simulink model "dummy2"  (R2018b)
settings: Solver=FixedStepDiscrete  StartTime=0.0  StopTime=10  FixedStep=0.2  RelTol=1e-3
undefined symbols (not defined in the file): eyen, n, xmin
settings Model: Creator=bradyplanden  LastModifiedBy=bradyplanden
settings OptimizationCC: DefaultParameterBehavior=Inlined
settings SFSimCC: SimCustomHeaderCode="#include \"dummy.h\""  SimUserSources=dummy.c  SimUserIncludeDirs=/usr/lib  SimUserLibraries=libblas.dylib liblapack.dylib  SimUseLocalCustomCode=off  SimAnalyzeCustomCode=on
settings RTWCC: GenerateReport=on  RTWUseLocalCustomCode=off  RTWUseSimCustomCode=on  CustomHeaderCode="#include \"dummy.h\""  CustomInclude=/usr/lib  CustomSource=dummy.c  CustomLibrary=libblas.dylib liblapack.dylib  LaunchReport=on
settings CodeAppCC: ForceParamTrailComments=on  StateflowObjectComments=on  MATLABSourceComments=on
settings GRTTargetCC: TargetLangStandard=C89/C90 (ANSI)

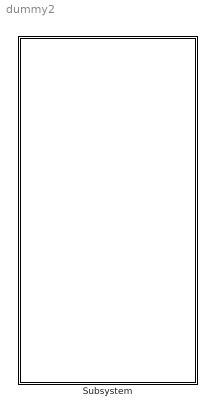
== system dummy2 ==
  Subsystem : Subsystem

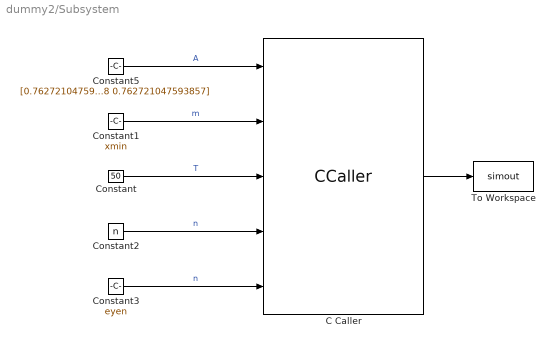
== system dummy2/Subsystem ==
  C Caller : CCaller  FunctionName=dummy2  PortSpecificationStruct="%)30     .    Z @   8    (     @         %    \"     8    !     0         %  0 \"0    $    V    07)G3F%M90  4&]R=$YA;64 4V-O<&4     26YD97@     5'EP90      4VEZ90         .    ,     8    (    !          %    \"     $    #     0         0  , ;W5T  X    P    !@    @    $          4    (     0    ,    !         !   P!O=70 #@   #@    &    \"     0         !0    @    !    !@    $         $     8   !/=7 ...(+2691 chars)"
  Constant : Constant  Value=50  OutDataTypeStr=Inherit: Inherit via back propagation  SampleTime=-1
  Constant1 : Constant  Value=xmin  OutDataTypeStr=Inherit: Inherit via back propagation  SampleTime=-1
  Constant2 : Constant  Value=n  OutDataTypeStr=Inherit: Inherit via back propagation  SampleTime=-1
  Constant3 : Constant  Value=eyen  OutDataTypeStr=Inherit: Inherit via back propagation  SampleTime=-1
  Constant5 : Constant  Value=|  OutDataTypeStr=Inherit: Inherit via back propagation  SampleTime=-1
      | [0.762721047593857	0.114882546593898	0.00247654474066823	2.09380749408769e-05	9.42229417535085e-08	2.63060135287668e-10	0.459613939727602	0.0198131117128797	0.000251260056028671	1.50757506761672e-06	5.26123024735364e-09	1.19993006342024e-11
      | 0.114882546593898	0.765197592334525	0.114903484668839	0.00247663896360998	2.09383380010122e-05	9.42229417535096e-08	0.0198131117128796	0.459865199783630	0.0198146192879473	0.000251265317258919	1.50758706691736e-06	5.26123024735407e-09
      | 0.00247654474066823	0.114903484668839	0.765197686557466	0.114903484931899	0.00247663896360999	2.09380749408770e-05	0.000251260056028671	0.0198146192879473	0.459865205044861	0.0198146192999466	0.000251265317258919	1.50757506761673e-06
      | 2.09380749408769e-05	0.00247663896360998	0.114903484931899	0.765197686557467	0.114903484668839	0.00247654474066823	1.50757506761672e-06	0.000251265317258918	0.0198146192999466	0.459865205044861	0.0198146192879473	0.000251260056028672
      | 9.42229417535087e-08	2.09383380010122e-05	0.00247663896360998	0.114903484668839	0.765197592334525	0.114882546593898	5.26123024735378e-09	1.50758706691736e-06	0.000251265317258919	0.0198146192879473	0.459865199783631	0.0198131117128796
      | 2.63060135287738e-10	9.42229417535093e-08	2.09380749408769e-05	0.00247654474066823	0.114882546593898	0.762721047593857	1.19993006342118e-11	5.26123024735394e-09	1.50757506761673e-06	0.000251260056028671	0.0198131117128797	0.459613939727602
      | -0.899414767742325	0.420238976357871	0.0193120991758899	0.000248250167123685	1.49706460642265e-06	5.23723164608530e-09	0.762721047593857	0.114882546593898	0.00247654474066823	2.09380749408769e-05	9.42229417535083e-08	2.63060135287700e-10
      | 0.420238976357871	-0.880102668566434	0.420487226524995	0.0193135962404963	0.000248255404355332	1.49706460642266e-06	0.114882546593898	0.765197592334525	0.114903484668839	0.00247663896360998	2.09383380010123e-05	9.42229417535099e-08
      | 0.0193120991758899	0.420487226524995	-0.880101171501828	0.420487231762227	0.0193135962404964	0.000248250167123686	0.00247654474066823	0.114903484668839	0.765197686557467	0.114903484931899	0.00247663896360999	2.09380749408770e-05
      | 0.000248250167123685	0.0193135962404963	0.420487231762227	-0.880101171501828	0.420487226524995	0.0193120991758899	2.09380749408769e-05	0.00247663896360998	0.114903484931899	0.765197686557467	0.114903484668839	0.00247654474066823
      | 1.49706460642265e-06	0.000248255404355331	0.0193135962404963	0.420487226524995	-0.880102668566434	0.420238976357871	9.42229417535088e-08	2.09383380010122e-05	0.00247663896360998	0.114903484668839	0.765197592334525	0.114882546593898
      | 5.23723164608547e-09	1.49706460642265e-06	0.000248250167123685	0.0193120991758899	0.420238976357872	-0.899414767742325	2.63060135287715e-10	9.42229417535098e-08	2.09380749408769e-05	0.00247654474066823	0.114882546593898	0.762721047593857]
  To Workspace : ToWorkspace  VariableName=simout  SaveFormat=Timeseries  SampleTime=-1
      settings: Decimation=4  Save2DSignal=2-D array (concatenate along first dimension)
  wires:
  Constant5/1 -> C Caller/1  "A"
  Constant2/1 -> C Caller/4  "n"
  Constant1/1 -> C Caller/2  "m"
  Constant/1 -> C Caller/3  "T"
  C Caller/1 -> To Workspace/1
  Constant3/1 -> C Caller/5  "n"
